simulink model "Task2_Indirect_MRAC"  (R2024b)
settings: Solver=ode45  StartTime=0.0  StopTime=120  MaxStep=0.01  RelTol=1e-7  AbsTol=1e-9
settings Model: Creator=LAPTOPASADI  LastModifiedBy=LAPTOPASADI
settings DataIOCC: SaveOutput=off  SignalLogging=off  SaveTime=off

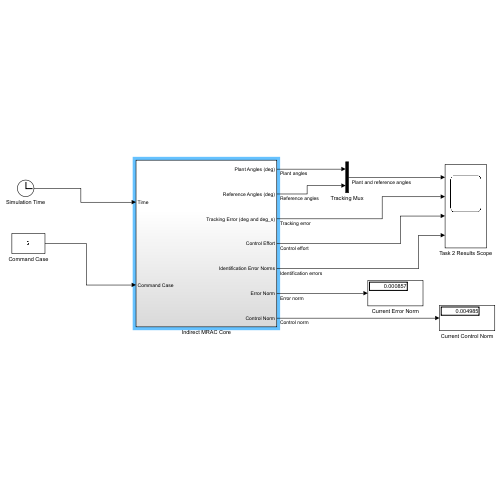
[thumbnail: Simulink's stored preview of the top-level diagram]
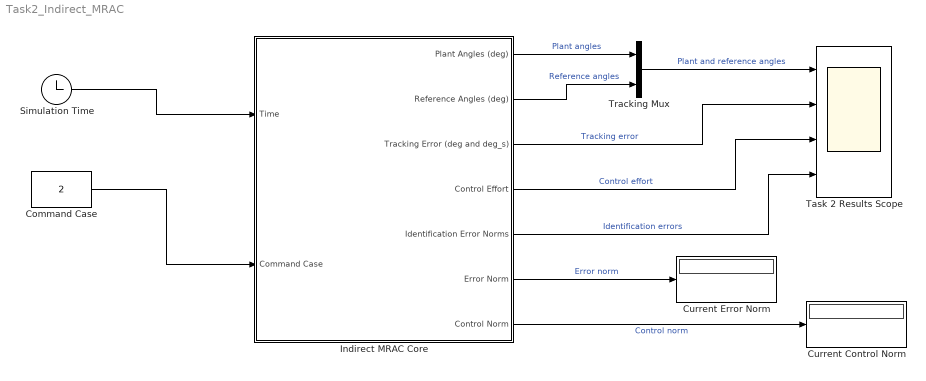
== system Task2_Indirect_MRAC ==
  Command Case : Constant  Value=2
  Current Control Norm : Display
  Current Error Norm : Display
  Indirect MRAC Core : Subsystem
  Simulation Time : Clock
  Task 2 Results Scope : Scope  NumInputPorts=4
  Tracking Mux : Mux  Inputs=2
  wires:
  Simulation Time/1 -> Indirect MRAC Core/1(Time)
  Command Case/1 -> Indirect MRAC Core/2(Command Case)
  Indirect MRAC Core/1(Plant Angles (deg)) -> Tracking Mux/1  "Plant angles"
  Indirect MRAC Core/2(Reference Angles (deg)) -> Tracking Mux/2  "Reference angles"
  Tracking Mux/1 -> Task 2 Results Scope/1  "Plant and reference angles"
  Indirect MRAC Core/3(Tracking Error (deg and deg_s)) -> Task 2 Results Scope/2  "Tracking error"
  Indirect MRAC Core/4(Control Effort) -> Task 2 Results Scope/3  "Control effort"
  Indirect MRAC Core/5(Identification Error Norms) -> Task 2 Results Scope/4  "Identification errors"
  Indirect MRAC Core/6(Error Norm) -> Current Error Norm/1  "Error norm"
  Indirect MRAC Core/7(Control Norm) -> Current Control Norm/1  "Control norm"

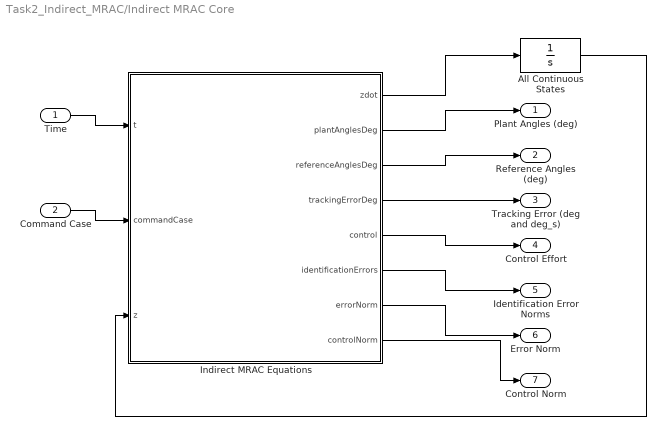
== system Task2_Indirect_MRAC/Indirect MRAC Core ==
  Time : Inport
  Command Case : Inport  Port=2
  All Continuous States : Integrator  InitialCondition=[0;0;0;0;0;0;0;0;0;0;0;0;0;0;0;0;0;0;1;0;0;0;0;0;0;0;0;0;1;0;0;0;0;0;0;0;0;0;1;0;0;0;0;0;0]
  Indirect MRAC Equations : MATLAB Function  TreatAsAtomicUnit=on
  Plant Angles (deg) : Outport
  Reference Angles (deg) : Outport  Port=2
  Tracking Error (deg and deg_s) : Outport  Port=3
  Control Effort : Outport  Port=4
  Identification Error Norms : Outport  Port=5
  Error Norm : Outport  Port=6
  Control Norm : Outport  Port=7
  wires:
  Time/1 -> Indirect MRAC Equations/1(t)
  Command Case/1 -> Indirect MRAC Equations/2(commandCase)
  All Continuous States/1 -> Indirect MRAC Equations/3(z)
  Indirect MRAC Equations/1(zdot) -> All Continuous States/1
  Indirect MRAC Equations/2(plantAnglesDeg) -> Plant Angles (deg)/1
  Indirect MRAC Equations/3(referenceAnglesDeg) -> Reference Angles (deg)/1
  Indirect MRAC Equations/4(trackingErrorDeg) -> Tracking Error (deg and deg_s)/1
  Indirect MRAC Equations/5(control) -> Control Effort/1
  Indirect MRAC Equations/6(identificationErrors) -> Identification Error Norms/1
  Indirect MRAC Equations/7(errorNorm) -> Error Norm/1
  Indirect MRAC Equations/8(controlNorm) -> Control Norm/1

== matlab function Task2_Indirect_MRAC/Indirect MRAC Core/Indirect MRAC Equations ==
  data: t input; zdot output; commandCase input; z input; plantAnglesDeg output; referenceAnglesDeg output; trackingErrorDeg output; control output; identificationErrors output; errorNorm output; controlNorm output
function [zdot,plantAnglesDeg,referenceAnglesDeg,trackingErrorDeg,control,identificationErrors,errorNorm,controlNorm] = indirectMRAC(t,commandCase,z)
%%#codegen
% Self-contained Task 2 model. No project .m file is called here.

x = z(1:6);
xm = z(7:12);
xPredictor = z(13:18);
WHat = reshape(z(19:45),9,3);

% Step or five-tone command. The command starts at one second.
reference = zeros(3,1);
if t >= 1
    if commandCase < 1.5
        reference = (pi/180)*[5;-5;8];
    else
        tau = t-1;
        weights = [0.30,0.24,0.19,0.15,0.12];
        peaks = (pi/180)*[10;10;15];
        amplitude = peaks*weights;
        frequency = [0.31,0.53,0.79,1.07,1.37; ...
                     0.37,0.61,0.89,1.19,1.43; ...
                     0.43,0.67,0.97,1.27,1.51];
        reference = sum(amplitude.*sin(frequency*tau),2);
    end
end

% Physical plant and reference-model matrices copied from Main.m.
dOverB = 1.2e-6/3.13e-5;
G = [0,0.175/0.0043,dOverB/0.0043; ...
     0.085/0.0142,0,0; ...
     0,dOverB/0.0176,-0.175/0.0176];
A = [zeros(3),eye(3);zeros(3),zeros(3)];
B = [zeros(3,3);G];
aP = (0.0142-0.0176)/0.0043;
aQ = (0.0176-0.0043)/0.0142;
aR = (0.0043-0.0142)/0.0176;
Htrue = [aP,0,0,-0.01,0,0; ...
         0,aQ,0,0,-0.01,0; ...
         0,0,aR,0,0,-0.01];
thetaPlantTrue = G\Htrue;
lambdaTrue = [0.80,0.05,0;0.05,1.10,0.03;0,0.03,0.90];

% Online estimates and regularized certainty-equivalence gains.
lambdaHat = WHat(1:3,:).';
thetaPlantHat = WHat(4:9,:).';
[U,S,V] = svd(lambdaHat);
singularValues = diag(S);
singularValues = max(singularValues,0.20);
lambdaInverse = V*diag(1./singularValues)*U.';
matchingState = G\[-4*eye(3),-4*eye(3)];
matchingReference = G\(4*eye(3));
KxHatT = lambdaInverse*matchingState;
KrHatT = lambdaInverse*matchingReference;
thetaHatT = lambdaInverse*thetaPlantHat;

p = x(4);
q = x(5);
rBody = x(6);
Phi = [q*rBody;p*rBody;p*q;p;q;rBody];
control = KxHatT*x + KrHatT*reference - thetaHatT*Phi;

% Plant, reference model, and series-parallel predictor.
xdot = A*x+B*(lambdaTrue*control+thetaPlantTrue*Phi);
xmdot = [xm(4:6);-4*xm(1:3)-4*xm(4:6)+4*reference];
omega = [control;Phi];
predictionError = x-xPredictor;
xPredictorDot = A*x+B*(WHat.'*omega)+4*predictionError;

% Gradient identifier: Gamma_W*omega*epsilon'*P_id*B.
identifierSignal = predictionError.'*(0.125*eye(6))*B;
gammaOmega = [200*omega(1:3);400*omega(4:9)];
WHatDot = gammaOmega*identifierSignal;
zdot = [xdot;xmdot;xPredictorDot;WHatDot(:)];

% Readable outputs for Scope and Display blocks only.
trackingError = x-xm;
plantAnglesDeg = (180/pi)*x(1:3);
referenceAnglesDeg = (180/pi)*xm(1:3);
trackingErrorDeg = (180/pi)*trackingError;
lambdaDifference = lambdaHat-lambdaTrue;
thetaDifference = thetaPlantHat-thetaPlantTrue;
identificationErrors = [sqrt(sum(predictionError.^2)); ...
                        sqrt(sum(lambdaDifference(:).^2)); ...
                        sqrt(sum(thetaDifference(:).^2))];
errorNorm = sqrt(sum(trackingError.^2));
controlNorm = sqrt(sum(control.^2));
end
